simulink model "Noeud"  (R2017a)
settings: Solver=VariableStepAuto  StartTime=0.0  StopTime=1  RelTol=1e-3
libraries: commrandsrc3 x1
settings Model: SimulationMode=accelerator  Creator=floriant  LastModifiedBy=floriant

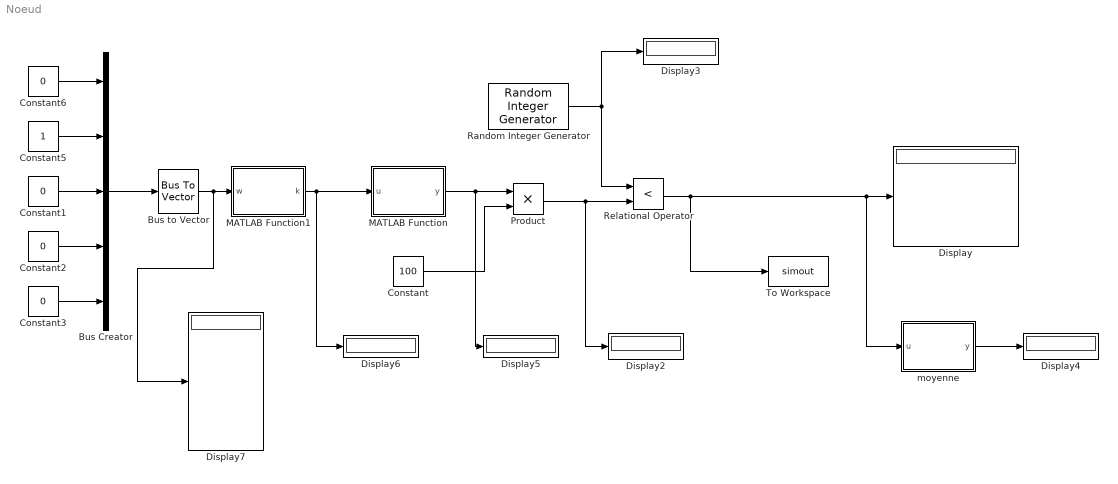
== system Noeud ==
  Bus Creator : BusCreator  Inputs=5
  Bus to Vector : BusToVector
  Constant : Constant  Value=100
  Constant{1..3,6} (4 alike) : Constant  Value=0  OutDataTypeStr=uint8
  Constant5 : Constant  OutDataTypeStr=uint8
  Display{,2..7} (7 alike) : Display
  MATLAB Function : MATLAB Function  TreatAsAtomicUnit=on
  MATLAB Function1 : MATLAB Function  TreatAsAtomicUnit=on
  Product : Product
  Random Integer Generator : commrandsrc3/Random Integer Generator  SetSize=100  SeedSource=Auto  Seed=0  SampleTime=1e-6  SamplesPerFrame=1  OutputDataType=uint8  SimulateUsing=Interpreted execution
  Relational Operator : RelationalOperator  Operator=<  OutDataTypeStr=boolean  RndMeth=Simplest
  To Workspace : ToWorkspace  VariableName=simout  SampleTime=-1
  moyenne : MATLAB Function  TreatAsAtomicUnit=on
  wires:
  Random Integer Generator/1 -> Relational Operator/1, Display3/1
  Relational Operator/1 -> To Workspace/1, moyenne/1(u), Display/1
  MATLAB Function/1(y) -> Display5/1, Product/1
  Product/1 -> Display2/1, Relational Operator/2
  Constant/1 -> Product/2
  moyenne/1(y) -> Display4/1
  MATLAB Function1/1(k) -> Display6/1, MATLAB Function/1(u)
  Bus to Vector/1 -> Display7/1, MATLAB Function1/1(w)
  Bus Creator/1 -> Bus to Vector/1
  Constant6/1 -> Bus Creator/1
  Constant5/1 -> Bus Creator/2
  Constant1/1 -> Bus Creator/3
  Constant2/1 -> Bus Creator/4
  Constant3/1 -> Bus Creator/5

== matlab function Noeud/moyenne ==
  data: u input; y output
function y = fcn(u)
persistent nb_one total
if isempty(nb_one)
    nb_one=0;
end
if isempty(total)
    total=0;
end
if u==1
    nb_one = nb_one+1;
end
total = total +1;

y=nb_one/total;

== matlab function Noeud/MATLAB Function ==
  data: u input; y output
function y = fcn(u)

MEM =[0.95;0.29;0.94;0.001];

y=MEM(u+1);

== matlab function Noeud/MATLAB Function1 ==
  data: w input; k output
function k = fcn(w)
out =0;
    if w(1)==1
        out = out + 1;
    end
    if w(2)==1
        out = out + 2;
    end
    if w(3)==1
        out = out + 4;
    end
    if w(4)==1
        out = out + 8;
    end
    if w(5)==1
        out = out + 16;
    end
k=out;
